simulink model "B4_quadcopter_model_discrete"  (R2021b)
settings: Solver=VariableStepAuto  StartTime=0.0  StopTime=10  FixedStep=0.002  RelTol=1e-3
values from neighbouring files (symbols this model uses):
  coef_sim_1 = tf_des_d.Denominator{1}(2)    [A11_setup_script_pprz.m]    (also in A1_setup_script.m; A6_slow_actuator.m)
  coef_sim_2 = tf_des_d.Numerator{1}(2)    [A11_setup_script_pprz.m]    (also in A1_setup_script.m; A6_slow_actuator.m)
  doublet_mag = - 0.15    (= -0.15)    [A11_setup_script_pprz.m]    (also in A1_setup_script.m)
  doublet_time = 6    [A11_setup_script_pprz.m]    (also in A1_setup_script.m)
  f_8 = 1    [A11_setup_script_pprz.m]    (also in A1_setup_script.m)
  FILT_CUTOFF = 2*pi*5    (= 31.4159265359)    [A11_setup_script_pprz.m]    (also in A1_setup_script.m)
  FILTER = 1    [A11_setup_script_pprz.m]    (also in A1_setup_script.m)
  G1 = inv(I)*G1_r    [A10_simple_plant.m]    (also in A11_setup_script_pprz.m = G1/scale; A1_setup_script.m = [G1;G1_T])
  G1_simple = inv(I)*G1_r_simple    [A1_setup_script.m]
  G2 = G2/scale    [A11_setup_script_pprz.m]    (also in A1_setup_script.m = (1/sampling_time)*inv(I)*(G2_r))
  h_plate = 0.3    [A11_setup_script_pprz.m]    (also in A1_setup_script.m = 0.16)
  I = eye(3,3)    [A10_simple_plant.m]    (also in A11_setup_script_pprz.m; A1_setup_script.m; A2_B_matrix_generation_symbolic.m = [Ixx 0 0; A3_B_matrix_generation_symbolic_cascaded.m = [Ixx 0 0)
  Iyy = 0.0008    [A11_setup_script_pprz.m]    (also in A1_setup_script.m = 0.0015)
  Izz = 0.000498    [A11_setup_script_pprz.m]    (also in A1_setup_script.m = 0.00015)
  K = 7    [A11_setup_script_pprz.m]    (also in A1_setup_script.m = 10)
  K_act = 50    [A10_simple_plant.m]    (also in A11_setup_script_pprz.m = 20; A1_setup_script.m = 20)
  K_act_outer = diag([K K K_act])    [A1_setup_script.m]
  K_d = 15    [A11_setup_script_pprz.m]    (also in A1_setup_script.m = 25)
  K_dd = K_act    (= 20)    [A11_setup_script_pprz.m]    (also in A1_setup_script.m)
  K_dyn = K    (= 10)    [A1_setup_script.m]
  K_ec = 50    [A11_setup_script_pprz.m]    (also in A1_setup_script.m = 251)
  K_ec_d = 13    [A11_setup_script_pprz.m]    (also in A1_setup_script.m = 25)
  K_ec_d_u = 1.5    [A11_setup_script_pprz.m]    (also in A1_setup_script.m = 5)
  K_ec_d_v = 1.5    [A11_setup_script_pprz.m]    (also in A1_setup_script.m = 5)
  K_ec_d_w = 1.5    [A11_setup_script_pprz.m]    (also in A1_setup_script.m = 5)
  K_ec_dd = 9    [A11_setup_script_pprz.m]    (also in A1_setup_script.m = 45)
  K_ec_i = 0    [A11_setup_script_pprz.m]    (also in A1_setup_script.m = 380)
  K_ec_u = 1.5    [A11_setup_script_pprz.m]    (also in A1_setup_script.m = 5)
  K_ec_v = 1.5    [A11_setup_script_pprz.m]    (also in A1_setup_script.m = 5)
  K_ec_w = 1.5    [A11_setup_script_pprz.m]    (also in A1_setup_script.m = 5)
  K_t = 0.0005    [A10_simple_plant.m]    (also in A11_setup_script_pprz.m = 6.557e-08; A1_setup_script.m = 6.557e-08)
  K_u = 1.0    (= 1)    [A11_setup_script_pprz.m]    (also in A1_setup_script.m = 1.5)
  K_u_d = 2.5    [A11_setup_script_pprz.m]    (also in A1_setup_script.m = 7)
  K_u_dd = K    (= 10)    [A1_setup_script.m]
  K_v = 1.0    (= 1)    [A11_setup_script_pprz.m]    (also in A1_setup_script.m = 1.5)
  K_v_d = 2.5    [A11_setup_script_pprz.m]    (also in A1_setup_script.m = 7)
  K_v_dd = K    (= 10)    [A1_setup_script.m]
  K_w = 1.0    (= 1)    [A11_setup_script_pprz.m]    (also in A1_setup_script.m = 4.5)
  K_w_d = 2.5    [A11_setup_script_pprz.m]    (also in A1_setup_script.m = 7)
  K_w_dd = K    (= 10)    [A1_setup_script.m]
  l_plate = 0.1    [A11_setup_script_pprz.m]    (also in A1_setup_script.m = 0.11)
  m = 0.4    [A10_simple_plant.m]    (also in A11_setup_script_pprz.m; A1_setup_script.m)
  NOISE = 0    [A11_setup_script_pprz.m]    (also in A1_setup_script.m)
  NOISE_ACC = 0.00005    (= 5e-05)    [A11_setup_script_pprz.m]    (also in A1_setup_script.m)
  NOISE_GYRO = 0.00005    (= 5e-05)    [A11_setup_script_pprz.m]    (also in A1_setup_script.m)
  NOISE_RPM = 200    [A11_setup_script_pprz.m]    (also in A1_setup_script.m)
  omega_act = 50    [A6_slow_actuator.m]
  omega_des = 20.00    (= 20)    [A11_setup_script_pprz.m]    (also in A1_setup_script.m; A6_slow_actuator.m = 49)
  sampling_time = 1/frequency    (= 0.002)    [A11_setup_script_pprz.m]    (also in A12_sim_multi_run.m; A1_setup_script.m; A6_slow_actuator.m)
  scale_8 = 1.6    [A11_setup_script_pprz.m]    (also in A1_setup_script.m)
  start_8 = 2    [A11_setup_script_pprz.m]    (also in A1_setup_script.m)
  start_time = 2    [A11_setup_script_pprz.m]    (also in A1_setup_script.m = 1)
  t_8 = 10    [A11_setup_script_pprz.m]    (also in A1_setup_script.m)
  w_plate = 0.3    [A11_setup_script_pprz.m]    (also in A1_setup_script.m = 0.36)
undefined symbols (not defined in the file or in its folder): DiscIntNeverNeededParam, K_ec_d_p, K_ec_d_q, K_ec_d_r, K_ec_dd_p, K_ec_dd_q, K_ec_dd_r, K_ec_i_u, K_ec_i_v, K_ec_i_w, K_ec_p, K_ec_q, K_ec_r, K_p, K_p_d, K_p_dd, K_q, K_q_d, K_q_dd, K_r, K_r_d, K_r_dd
libraries: simulink x44, cstblocks x37, dspinverses x26, dspmathops x9, dspstat3 x9, aerolibutil x9, sharedutil x3, aerolibanim x1
(part 4 of 13)

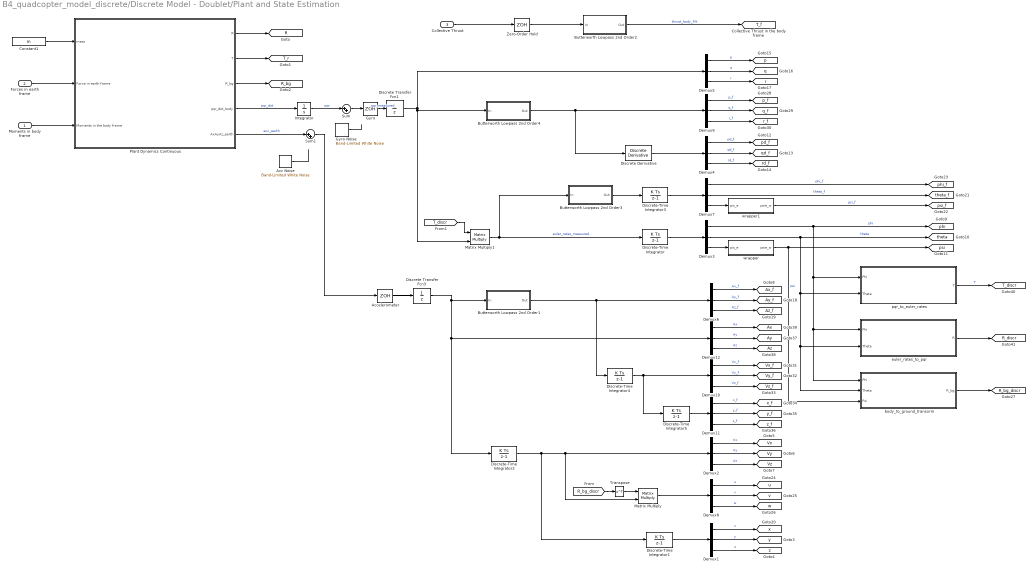
== system B4_quadcopter_model_discrete/Discrete Model - Doublet/Plant and State Estimation ==
  Moments in body frame : Inport
  Forces in earth frame : Inport  Port=2
  Collective Thrust : Inport  Port=3
  Acc Noise : simulink/Sources/Band-Limited White Noise  Cov=[NOISE_ACC]  Ts=sampling_time  seed=[23341]
  Accelerometer : ZeroOrderHold  SampleTime=sampling_time
  Butterworth Lowpass 2nd Order1 : Subsystem
  Butterworth Lowpass 2nd Order2 : Subsystem
  Butterworth Lowpass 2nd Order3 : Subsystem
  Butterworth Lowpass 2nd Order4 : Subsystem
  Constant1 : Constant  Value=m  SampleTime=sampling_time
  Demux{1..12} (12 alike) : Demux  Outputs=3
  Discrete Transfer Fcn1 : DiscreteTransferFcn  Denominator=[1 0]
  Discrete Transfer Fcn3 : DiscreteTransferFcn  Denominator=[1 0]
  Discrete Derivative : simulink/Discrete/Discrete Derivative  gainval=1.0  ICPrevScaledInput=0.0  OutMin=[]  OutMax=[]  OutDataType=fixdt(1, 16)  OutScaling=2^-10  DoSatur=off
  Discrete-Time Integrator{,1..5} (6 alike) : DiscreteIntegrator  SampleTime=sampling_time  ICPrevOutput=DiscIntNeverNeededParam  ICPrevScaledInput=DiscIntNeverNeededParam
  Gyro : ZeroOrderHold  SampleTime=sampling_time
  Gyro Noise : simulink/Sources/Band-Limited White Noise  Cov=[NOISE_GYRO]  Ts=sampling_time  seed=[23341]
  Integrator : Integrator
  Matrix Multiply : Product  Multiplication=Matrix(*)
  Matrix Multiply1 : Product  Multiplication=Matrix(*)
  Plant Dynamics Continuous : Subsystem
  Sum : Sum  Inputs=|++
  Sum1 : Sum  Inputs=|++
  Transpose : Math  Operator=transpose  SaturateOnIntegerOverflow=on
  Zero-Order Hold : ZeroOrderHold  SampleTime=sampling_time
  body_to_ground_transorm : MATLAB Function  Description=|  TreatAsAtomicUnit=on
      | This function computes the rotational matrix to pass from the body frame to the world frame. 
      | Takes as inpout the euler angles.
  euler_rates_to_pqr : MATLAB Function  TreatAsAtomicUnit=on
  pqr_to_euler_rates : MATLAB Function  TreatAsAtomicUnit=on
  wrapper : MATLAB Function  TreatAsAtomicUnit=on
  wrapper1 : MATLAB Function  TreatAsAtomicUnit=on
  tag scope: Ax=global, Ax_f=global, Ay=global, Ay_f=global, Az=global, Az_f=global, R=global, R_bg=global, R_bg_discr=global, R_discr=global, T_discr=global, T_f=global, T_r=global, Vx=global, Vx_f=global, Vy=global, Vy_f=global, Vz=global, Vz_f=global, p=global, p_f=global, pd_f=global, phi=global, phi_f=global, psi=global, psi_f=global, q=global, q_f=global, qd_f=global, r=global, r_f=global, rd_f=global, theta=global, theta_f=global, u=global, v=global, w=global, x=global, x_f=global, y=global, y_f=global, z=global, z_f=global
  wires:
  Demux3/2 -> body_to_ground_transorm/2(Theta), euler_rates_to_pqr/2(Theta), pqr_to_euler_rates/2(Theta), [theta]  "theta"
  Demux4/1 -> [pd_f]  "pd_f"
  Demux3/1 -> body_to_ground_transorm/1(Phi), euler_rates_to_pqr/1(Phi), pqr_to_euler_rates/1(Phi), [phi]  "phi"
  Demux4/2 -> [qd_f]  "qd_f"
  Demux3/3 -> wrapper/1(pis_e)
  Discrete-Time Integrator/1 -> Demux3/1
  Demux5/2 -> [q]  "q"
  Demux5/1 -> [p]  "p"
  Plant Dynamics Continuous/4(pqr_dot_body) -> Integrator/1  "pqr_dot"
  Demux5/3 -> [r]  "r"
  Integrator/1 -> Sum/1  "pqr"
  Demux4/3 -> [rd_f]  "rd_f"
  Moments in body frame/1 -> Plant Dynamics Continuous/3(Moments in the body frame)
  Constant1/1 -> Plant Dynamics Continuous/1(mass)
  Forces in earth frame/1 -> Plant Dynamics Continuous/2(Force in earth frame)
  Plant Dynamics Continuous/1(R) -> [R]
  Plant Dynamics Continuous/2(T) -> [T_r]
  Plant Dynamics Continuous/3(R_bg) -> [R_bg]
  Demux2/2 -> [Vy]  "Vy"
  Demux6/2 -> [Ay_f]  "Ay_f"
  Discrete-Time Integrator1/1 -> Demux1/1
  Demux6/1 -> [Ax_f]  "Ax_f"
  Accelerometer/1 -> Discrete Transfer Fcn3/1
  Demux2/1 -> [Vx]  "Vx"
  Demux1/2 -> [y]  "y"
  Demux1/1 -> [x]  "x"
  Demux1/3 -> [z]  "z"
  Demux6/3 -> [Az_f]  "Az_f"
  Discrete-Time Integrator2/1 -> Demux2/1, Matrix Multiply/2, Discrete-Time Integrator1/1
  Demux2/3 -> [Vz]  "Vz"
  Plant Dynamics Continuous/5(AxAyAz_earth) -> Sum1/1  "acc_earth"
  Demux7/3 -> wrapper1/1(pis_e)
  Demux7/1 -> [phi_f]  "phi_f"
  Demux7/2 -> [theta_f]  "theta_f"
  Discrete-Time Integrator3/1 -> Demux7/1
  [R_bg_discr] -> Transpose/1
  Transpose/1 -> Matrix Multiply/1
  Demux8/2 -> [v]  "v"
  Demux8/1 -> [u]  "u"
  Demux8/3 -> [w]  "w"
  Matrix Multiply/1 -> Demux8/1
  Gyro/1 -> Discrete Transfer Fcn1/1  "pqr_measured"
  Zero-Order Hold/1 -> Butterworth Lowpass 2nd Order2/1(In)
  Butterworth Lowpass 2nd Order2/1(Out) -> [T_f]  "thrust_body_filt"
  Collective Thrust/1 -> Zero-Order Hold/1
  Demux9/3 -> [r_f]  "r_f"
  Demux9/1 -> [p_f]  "p_f"
  Demux9/2 -> [q_f]  "q_f"
  Demux10/1 -> [Vx_f]  "Vx_f"
  Demux10/2 -> [Vy_f]  "Vy_f"
  Demux10/3 -> [Vz_f]  "Vz_f"
  Demux11/2 -> [y_f]  "y_f"
  Discrete-Time Integrator5/1 -> Demux11/1
  Demux11/1 -> [x_f]  "x_f"
  Demux11/3 -> [z_f]  "z_f"
  Discrete-Time Integrator4/1 -> Discrete-Time Integrator5/1, Demux10/1
  Demux12/2 -> [Ay]  "Ay"
  Demux12/1 -> [Ax]  "Ax"
  Demux12/3 -> [Az]  "Az"
  [T_discr] -> Matrix Multiply1/1
  Matrix Multiply1/1 -> Butterworth Lowpass 2nd Order3/1(In), Discrete-Time Integrator/1  "euler_rates_measured"
  Butterworth Lowpass 2nd Order3/1(Out) -> Discrete-Time Integrator3/1
  euler_rates_to_pqr/1(R) -> [R_discr]
  pqr_to_euler_rates/1(T) -> [T_discr]  "T"
  body_to_ground_transorm/1(R_bg) -> [R_bg_discr]
  Butterworth Lowpass 2nd Order1/1(Out) -> Demux6/1, Discrete-Time Integrator4/1
  wrapper/1(psie_w) -> body_to_ground_transorm/3(Psi), [psi]  "psi"
  wrapper1/1(psie_w) -> [psi_f]  "psi_f"
  Sum/1 -> Gyro/1
  Gyro Noise/1 -> ?
  Acc Noise/1 -> ?
  Sum1/1 -> Accelerometer/1
  Discrete Transfer Fcn1/1 -> Demux5/1, Butterworth Lowpass 2nd Order4/1(In), Matrix Multiply1/2
  Discrete Derivative/1 -> Demux4/1
  Discrete Transfer Fcn3/1 -> Discrete-Time Integrator2/1, Demux12/1, Butterworth Lowpass 2nd Order1/1(In)
  Butterworth Lowpass 2nd Order4/1(Out) -> Demux9/1, Discrete Derivative/1

== system B4_quadcopter_model_discrete/Discrete Model - Inner Loop Only/Continuous Actuator Dynamics ==
  Motor_1_omega_input : Inport
  Motor_2_omega_input : Inport  Port=2
  Motor_3_omega_input : Inport  Port=3
  Motor_4_omega_input : Inport  Port=4
  Butterworth Lowpass 2nd Order1 : Subsystem
  Demux : Demux
  Discrete Transfer Fcn{1..4} (4 alike) : DiscreteTransferFcn  Numerator=[coef_sim_2]  Denominator=[1 coef_sim_1]  SampleTime=sampling_time
  Mux : Mux
  RPM Noise : simulink/Sources/Band-Limited White Noise  Cov=[NOISE_RPM]  Ts=sampling_time  seed=[23341]
  Saturation{,1..3} (4 alike) : Saturate  UpperLimit=12000  LowerLimit=0
  Sum : Sum  Inputs=|++
  Transfer Fcn{,1..3} (4 alike) : TransferFcn  Numerator=[omega_des]  Denominator=[1 omega_des]
  omega_1 : Outport
  omega_2 : Outport  Port=2
  omega_3 : Outport  Port=3
  omega_4 : Outport  Port=4
  tag scope: omega_1_f=global, omega_2_f=global, omega_3_f=global, omega_4_f=global
  wires:
  Transfer Fcn3/1 -> omega_4/1  "omega_4"
  Motor_4_omega_input/1 -> Saturation3/1  "omega_4_in"
  Saturation/1 -> Discrete Transfer Fcn2/1, Transfer Fcn/1
  Motor_3_omega_input/1 -> Saturation2/1  "omega_3_in"
  Transfer Fcn1/1 -> omega_2/1  "omega_2"
  Saturation1/1 -> Transfer Fcn1/1, Discrete Transfer Fcn1/1
  Saturation3/1 -> Transfer Fcn3/1, Discrete Transfer Fcn4/1
  Discrete Transfer Fcn2/1 -> Mux/1
  Saturation2/1 -> Transfer Fcn2/1, Discrete Transfer Fcn3/1
  Motor_2_omega_input/1 -> Saturation1/1  "omega_2_in"
  Demux/2 -> [omega_2_f]  "omega_2_est"
  Motor_1_omega_input/1 -> Saturation/1  "omega_1_in"
  Transfer Fcn/1 -> omega_1/1  "omega_1"
  Demux/4 -> [omega_4_f]  "omega_4_est"
  Discrete Transfer Fcn4/1 -> Mux/4
  Discrete Transfer Fcn1/1 -> Mux/2
  Discrete Transfer Fcn3/1 -> Mux/3
  Transfer Fcn2/1 -> omega_3/1  "omega_3"
  Demux/1 -> [omega_1_f]  "omega_1_est"
  Demux/3 -> [omega_3_f]  "omega_3_est"
  Mux/1 -> Sum/1
  Butterworth Lowpass 2nd Order1/1(Out) -> Demux/1
  RPM Noise/1 -> ?
  Sum/1 -> Butterworth Lowpass 2nd Order1/1(In)

== system B4_quadcopter_model_discrete/Discrete Model - Inner Loop Only/Discrete INDI Controller Cascaded ==
  note: Inner Loop
  Constant : Constant  Value=0
  Constant2 : Constant  Value=G1  SampleTime=sampling_time
  Constant3 : Constant  Value=G2  SampleTime=sampling_time
  Constant9 : Constant  Value=G2  SampleTime=sampling_time
  Demux : Demux
  Demux1 : Demux  Outputs=3
  Discrete Transfer Fcn : DiscreteTransferFcn  Denominator=[1 0]
  Display : Display
  Doublet Block : Subsystem
  ERROR CONTROLLER ATTITUDE : Subsystem
  G1+G2 : MATLAB Function  TreatAsAtomicUnit=on
  G2_comp : MATLAB Function  TreatAsAtomicUnit=on
  INTERNAL REFERENCE MODEL ATTITUDE : Subsystem
  Matrix Multiply : Product  Multiplication=Matrix(*)
  Pseudoinverse2 : dspinverses/Pseudoinverse  wanterr=off  SimulateUsing=Interpreted execution
      settings: SourceProductBaseCode=DS
  Saturation4 : Saturate  UpperLimit=12000  LowerLimit=10
  Scope1 : Scope
  Sum{,4..5,8,11,13} (6 alike) : Sum  Inputs=|++
  Sum1 : Sum  Inputs=|+-
  Sum2 : Sum  Inputs=|+-
  Sum3 : Sum  Inputs=|+-
  Vector Concatenate : Concatenate  NumInputs=3
  Vector Concatenate1 : Concatenate  NumInputs=4
  Vector Concatenate2 : Concatenate  NumInputs=3
  Motor_1_omega_input : Outport
  Motor_2_omega_input : Outport  Port=2
  Motor_3_omega_input : Outport  Port=3
  Motor_4_omega_input : Outport  Port=4
  wires:
  Sum13/1 -> Sum3/1  "rd_des"
  Sum4/1 -> Sum1/1  "pd_des"
  Sum2/1 -> Vector Concatenate/2
  ERROR CONTROLLER ATTITUDE/1(pd_ec) -> Sum4/2  "pd_ec"
  Sum3/1 -> Vector Concatenate/3
  ERROR CONTROLLER ATTITUDE/3(rd_ec) -> Sum13/2  "rd_ec"
  INTERNAL REFERENCE MODEL ATTITUDE/5(q_ref) -> ERROR CONTROLLER ATTITUDE/2(q_ref)  "q_ref"
  Vector Concatenate/1 -> [dv_inner], Scope1/1
  [pd_f] -> Sum1/2
  INTERNAL REFERENCE MODEL ATTITUDE/3(rd_ref) -> Sum13/1  "rd_ref"
  INTERNAL REFERENCE MODEL ATTITUDE/9(psi_ref) -> ERROR CONTROLLER ATTITUDE/6(psi_ref)  "psi_ref"
  INTERNAL REFERENCE MODEL ATTITUDE/4(p_ref) -> ERROR CONTROLLER ATTITUDE/1(p_ref)  "p_ref"
  INTERNAL REFERENCE MODEL ATTITUDE/6(r_ref) -> ERROR CONTROLLER ATTITUDE/3(r_ref)  "r_ref"
  INTERNAL REFERENCE MODEL ATTITUDE/8(theta_ref) -> ERROR CONTROLLER ATTITUDE/5(theta_ref)  "theta_ref"
  INTERNAL REFERENCE MODEL ATTITUDE/7(phi_ref) -> ERROR CONTROLLER ATTITUDE/4(phi_ref)  "phi_ref"
  ERROR CONTROLLER ATTITUDE/2(qd_ec) -> Sum11/2  "qd_ec"
  INTERNAL REFERENCE MODEL ATTITUDE/1(pd_ref) -> Sum4/1  "pd_ref"
  Sum1/1 -> Vector Concatenate/1
  Sum11/1 -> Sum2/1  "qd_des"
  [qd_f] -> Sum2/2
  INTERNAL REFERENCE MODEL ATTITUDE/2(qd_ref) -> Sum11/1  "qd_ref"
  [rd_f] -> Sum3/2
  Saturation4/1 -> Discrete Transfer Fcn/1
  Demux/4 -> Motor_4_omega_input/1
  Pseudoinverse2/1 -> Matrix Multiply/1
  Vector Concatenate2/1 -> Matrix Multiply/2
  Constant9/1 -> G2_comp/1(G2)
  Sum/1 -> Vector Concatenate2/3
  Demux1/3 -> Sum/1
  Demux1/2 -> Vector Concatenate2/2
  Constant2/1 -> G1+G2/1(G1)
  Discrete Transfer Fcn/1 -> G2_comp/2(domega)
  Constant3/1 -> G1+G2/2(G2)
  Demux/3 -> Motor_3_omega_input/1
  [omega_1_f] -> Vector Concatenate1/1
  Vector Concatenate1/1 -> Sum8/2  "u"
  G2_comp/1(G2_comp) -> Sum/2  "G2_comp"
  Demux1/1 -> Vector Concatenate2/1
  Matrix Multiply/1 -> Saturation4/1, Sum8/1  "du"
  Demux/1 -> Motor_1_omega_input/1
  [omega_3_f] -> Vector Concatenate1/3
  Sum8/1 -> Demux/1  "u_cmd"
  Demux/2 -> Motor_2_omega_input/1
  [omega_2_f] -> Vector Concatenate1/2
  G1+G2/1(B_inner) -> Pseudoinverse2/1, Display/1  "B_inner"
  [dv_inner] -> Demux1/1  "dv_inner"
  [omega_4_f] -> Vector Concatenate1/4
  Constant/1 -> INTERNAL REFERENCE MODEL ATTITUDE/1(phi_cmd), Sum5/1  "phi_cmd"
  Sum5/1 -> INTERNAL REFERENCE MODEL ATTITUDE/2(theta_cmd)  "theta_cmd"
  Doublet Block/1(Out1) -> Sum5/2

== system B4_quadcopter_model_discrete/Discrete Model - Inner Loop Only/Discrete INDI Controller Cascaded w// Actuator Compensation ==
  Constant : Constant  Value=0
  Constant2 : Constant  Value=G1_simple  SampleTime=sampling_time
  Constant6 : Constant  Value=K_act  SampleTime=sampling_time
  Demux : Demux
  Display : Display
  Doublet Block : Subsystem
  ERROR CONTROLLER ATTITUDE : Subsystem
  G1+G2 : MATLAB Function  TreatAsAtomicUnit=on
  INTERNAL REFERENCE MODEL ATTITUDE : Subsystem
  Matrix Multiply : Product  Multiplication=Matrix(*)
  Pseudoinverse2 : dspinverses/Pseudoinverse  wanterr=off  SimulateUsing=Interpreted execution
      settings: SourceProductBaseCode=DS
  Sum{1,4,8,11,13} (5 alike) : Sum  Inputs=|++
  Vector Concatenate : Concatenate  NumInputs=3
  Vector Concatenate1 : Concatenate  NumInputs=4
  Motor_1_omega_input : Outport
  Motor_2_omega_input : Outport  Port=2
  Motor_3_omega_input : Outport  Port=3
  Motor_4_omega_input : Outport  Port=4
  wires:
  G1+G2/1(B_inner) -> Pseudoinverse2/1, Display/1  "B_inner"
  Vector Concatenate1/1 -> Sum8/2  "u"
  Vector Concatenate/1 -> [dv_inner]
  Matrix Multiply/1 -> Sum8/1  "du"
  Demux/1 -> Motor_1_omega_input/1
  [omega_4_f] -> Vector Concatenate1/4
  [omega_2_f] -> Vector Concatenate1/2
  Demux/3 -> Motor_3_omega_input/1
  Sum8/1 -> Demux/1  "u_cmd"
  Pseudoinverse2/1 -> Matrix Multiply/1
  [omega_1_f] -> Vector Concatenate1/1
  Demux/2 -> Motor_2_omega_input/1
  Demux/4 -> Motor_4_omega_input/1
  [omega_3_f] -> Vector Concatenate1/3
  INTERNAL REFERENCE MODEL ATTITUDE/4(pd_ref) -> ERROR CONTROLLER ATTITUDE/1(pd_ref)
  INTERNAL REFERENCE MODEL ATTITUDE/7(p_ref) -> ERROR CONTROLLER ATTITUDE/4(p_ref)
  ERROR CONTROLLER ATTITUDE/3(rdd_ec) -> Sum13/2  "rdd_ec"
  ERROR CONTROLLER ATTITUDE/2(qdd_ec) -> Sum11/2  "qdd_ec"
  INTERNAL REFERENCE MODEL ATTITUDE/5(qd_ref) -> ERROR CONTROLLER ATTITUDE/2(qd_ref)
  INTERNAL REFERENCE MODEL ATTITUDE/11(theta_ref) -> ERROR CONTROLLER ATTITUDE/8(theta_ref)
  INTERNAL REFERENCE MODEL ATTITUDE/1(pdd_ref) -> Sum4/1
  INTERNAL REFERENCE MODEL ATTITUDE/3(rdd_ref) -> Sum13/1
  INTERNAL REFERENCE MODEL ATTITUDE/8(q_ref) -> ERROR CONTROLLER ATTITUDE/5(q_ref)
  ERROR CONTROLLER ATTITUDE/1(pdd_ec) -> Sum4/2  "pdd_ec"
  INTERNAL REFERENCE MODEL ATTITUDE/6(rd_ref) -> ERROR CONTROLLER ATTITUDE/3(rd_ref)
  INTERNAL REFERENCE MODEL ATTITUDE/10(phi_ref) -> ERROR CONTROLLER ATTITUDE/7(phi_ref)
  INTERNAL REFERENCE MODEL ATTITUDE/12(psi_ref) -> ERROR CONTROLLER ATTITUDE/9(psi_ref)
  INTERNAL REFERENCE MODEL ATTITUDE/9(r_ref) -> ERROR CONTROLLER ATTITUDE/6(r_ref)
  Sum13/1 -> Vector Concatenate/3  "rdd_des"
  Sum4/1 -> Vector Concatenate/1  "pdd_des"
  Sum11/1 -> Vector Concatenate/2  "qdd_des"
  Constant6/1 -> G1+G2/2(K_act)
  Constant2/1 -> G1+G2/1(G1_simple)
  [dv_inner] -> Matrix Multiply/2  "dv_inner"
  INTERNAL REFERENCE MODEL ATTITUDE/2(qdd_ref) -> Sum11/1
  Constant/1 -> INTERNAL REFERENCE MODEL ATTITUDE/3(psi_cmd), INTERNAL REFERENCE MODEL ATTITUDE/1(phi_cmd), Sum1/1  "phi_cmd"
  Sum1/1 -> INTERNAL REFERENCE MODEL ATTITUDE/2(theta_cmd)  "theta_cmd"
  Doublet Block/1(Out1) -> Sum1/2

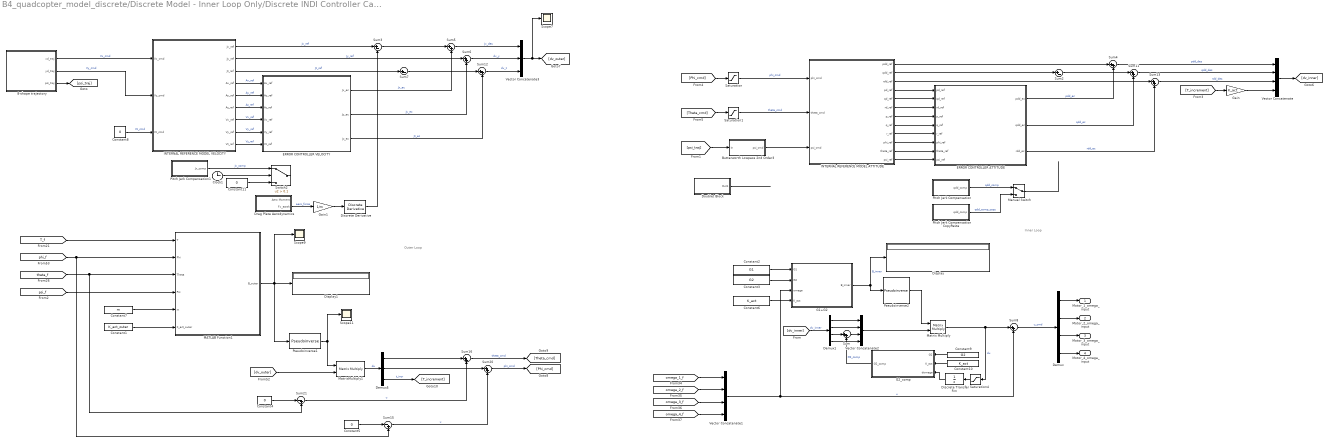
== system B4_quadcopter_model_discrete/Discrete Model - Inner Loop Only/Discrete INDI Controller Cascaded w// Actuator Compensation Double ==
  note: Outer Loop
  note: Inner Loop
  8-shape trajectory : Subsystem
  Butterworth Lowpass 2nd Order3 : Subsystem
  Clock1 : Clock
      settings: Decimation=100
  Constant1 : Constant  Value=K_act_outer  SampleTime=sampling_time
  Constant10 : Constant  Value=K_act  SampleTime=sampling_time
  Constant11 : Constant  Value=0
  Constant2 : Constant  Value=G1  SampleTime=sampling_time
  Constant3 : Constant  Value=G2  SampleTime=sampling_time
  Constant4 : Constant  Value=0
  Constant5 : Constant  Value=0
  Constant6 : Constant  Value=K_act  SampleTime=sampling_time
  Constant7 : Constant  Value=m  SampleTime=sampling_time
  Constant8 : Constant  Value=0  SampleTime=sampling_time
  Constant9 : Constant  Value=G2  SampleTime=sampling_time
  Demux : Demux
  Demux1 : Demux
  Demux5 : Demux  Outputs=3
  Discrete Transfer Fcn : DiscreteTransferFcn  Denominator=[1 0]
  Discrete Derivative : simulink/Discrete/Discrete Derivative  gainval=1.0  ICPrevScaledInput=0.0  OutMin=[]  OutMax=[]  OutDataType=fixdt(1, 16)  OutScaling=2^-10  DoSatur=off
  Display : Display
  Display1 : Display
  Doublet Block : Subsystem
  Drag Plate Aerodynamics : Subsystem
  ERROR CONTROLLER ATTITUDE : Subsystem
  ERROR CONTROLLER VELOCITY : Subsystem
  G1+G2 : MATLAB Function  TreatAsAtomicUnit=on
  G2_comp : MATLAB Function  TreatAsAtomicUnit=on
  Gain : Gain  Gain=K_act
  Gain1 : Gain  Gain=1/m
  INTERNAL REFERENCE MODEL ATTITUDE : Subsystem
  INTERNAL REFERENCE MODEL VELOCITY : Subsystem
  MATLAB Function1 : MATLAB Function  TreatAsAtomicUnit=on
  Manual Switch : ManualSwitch
  Matrix Multiply : Product  Multiplication=Matrix(*)
  MatrixMultiply1 : Product  Multiplication=Matrix(*)
  Pitch Jerk Compensation : Subsystem
  Pitch Jerk Compensation CopyPaste : Subsystem
  Pitch Jerk Compensation1 : Subsystem
  Pseudoinverse1 : dspinverses/Pseudoinverse  wanterr=off  SimulateUsing=Interpreted execution
      settings: SourceProductBaseCode=DS
  Pseudoinverse2 : dspinverses/Pseudoinverse  wanterr=off  SimulateUsing=Interpreted execution
      settings: SourceProductBaseCode=DS
  Saturation : Saturate
  Saturation1 : Saturate
  Saturation4 : Saturate  UpperLimit=12000  LowerLimit=10
  Scope11 : Scope
  Scope7 : Scope
  Scope9 : Scope
  Sum{,4..6,8,11..13,16,20} (10 alike) : Sum  Inputs=|++
  Sum15 : Sum  Inputs=|-+
  Sum2 : Sum  Inputs=|+-
  Sum21 : Sum  Inputs=|-+
  Sum3 : Sum  Inputs=|+-
  Sum7 : Sum  Inputs=|+-
  Switch2 : Switch  Criteria=u2 > Threshold  Threshold=0.1
  Vector Concatenate : Concatenate  NumInputs=4
  Vector Concatenate1 : Concatenate  NumInputs=4
  Vector Concatenate2 : Concatenate  NumInputs=4
  Vector Concatenate3 : Concatenate  NumInputs=3
  Motor_1_omega_input : Outport
  Motor_2_omega_input : Outport  Port=2
  Motor_3_omega_input : Outport  Port=3
  Motor_4_omega_input : Outport  Port=4
  wires:
  Constant4/1 -> Sum21/1
  Sum16/1 -> [Theta_cmd]  "theta_cmd"
  Sum12/1 -> Vector Concatenate3/3  "dv_z"
  INTERNAL REFERENCE MODEL VELOCITY/2(Jy_ref) -> Sum6/1  "Jy_ref"
  Sum21/1 -> Sum16/2  "u"
  ERROR CONTROLLER VELOCITY/2(Jy_ec) -> Sum6/2  "Jy_ec"
  8-shape trajectory/1(xd_traj) -> INTERNAL REFERENCE MODEL VELOCITY/1(Vx_cmd)  "Vx_cmd"
  Sum6/1 -> Vector Concatenate3/2  "dv_y"
  ERROR CONTROLLER VELOCITY/1(Jx_ec) -> Sum5/2  "Jx_ec"
  Sum5/1 -> Vector Concatenate3/1  "Jx_des"
  ERROR CONTROLLER VELOCITY/3(Jz_ec) -> Sum12/2  "Jz_ec"
  Constant8/1 -> INTERNAL REFERENCE MODEL VELOCITY/3(Vz_cmd)  "Vz_cmd"
  Pseudoinverse1/1 -> Scope11/1, MatrixMultiply1/1
  Sum15/1 -> Sum20/2  "u"
  Vector Concatenate3/1 -> Scope7/1, [dv_outer]
  INTERNAL REFERENCE MODEL VELOCITY/1(Jx_ref) -> Sum3/1  "Jx_ref"
  INTERNAL REFERENCE MODEL VELOCITY/3(Jz_ref) -> Sum7/1  "Jz_ref"
  Sum20/1 -> [Phi_cmd]  "phi_cmd"
  [T_f] -> MATLAB Function1/1(T)
  Constant7/1 -> MATLAB Function1/5(m)
  Constant5/1 -> Sum15/1
  [dv_outer] -> MatrixMultiply1/2
  Demux5/1 -> Sum16/1
  MATLAB Function1/1(B_outer) -> Pseudoinverse1/1, Display1/1, Scope9/1
  Demux5/3 -> [T_increment]  "t_incr"
  MatrixMultiply1/1 -> Demux5/1  "du"
  Demux5/2 -> Sum20/1
  8-shape trajectory/2(yd_traj) -> INTERNAL REFERENCE MODEL VELOCITY/2(Vy_cmd)  "Vy_cmd"
  [theta_f] -> Sum21/2, MATLAB Function1/3(Theta)
  [phi_f] -> Sum15/2, MATLAB Function1/2(Phi)
  8-shape trajectory/3(psi_traj) -> [psi_traj]
  INTERNAL REFERENCE MODEL VELOCITY/4(Ax_ref) -> ERROR CONTROLLER VELOCITY/1(Ax_ref)  "Ax_ref"
  INTERNAL REFERENCE MODEL VELOCITY/5(Ay_ref) -> ERROR CONTROLLER VELOCITY/2(Ay_ref)  "Ay_ref"
  INTERNAL REFERENCE MODEL VELOCITY/6(Az_ref) -> ERROR CONTROLLER VELOCITY/3(Az_ref)  "Az_ref"
  INTERNAL REFERENCE MODEL VELOCITY/7(Vx_ref) -> ERROR CONTROLLER VELOCITY/4(Vx_ref)  "Vx_ref"
  INTERNAL REFERENCE MODEL VELOCITY/8(Vy_ref) -> ERROR CONTROLLER VELOCITY/5(Vy_ref)  "Vy_ref"
  INTERNAL REFERENCE MODEL VELOCITY/9(Vz_ref) -> ERROR CONTROLLER VELOCITY/6(Vz_ref)  "Vz_ref"
  Sum3/1 -> Sum5/1
  Sum7/1 -> Sum12/1
  Constant1/1 -> MATLAB Function1/6(K_act_outer)
  [psi_f] -> MATLAB Function1/4(Psi)
  INTERNAL REFERENCE MODEL ATTITUDE/12(psi_ref) -> ERROR CONTROLLER ATTITUDE/9(psi_ref)
  Demux1/1 -> Vector Concatenate2/1
  ERROR CONTROLLER ATTITUDE/2(qdd_ec) -> Sum11/2  "qdd_ec"
  Sum4/1 -> Vector Concatenate/1  "pdd_des"
  [dv_inner] -> Demux1/1  "dv_inner"
  Demux1/4 -> Vector Concatenate2/4
  INTERNAL REFERENCE MODEL ATTITUDE/3(rdd_ref) -> Sum13/1
  Sum2/1 -> Sum11/1
  INTERNAL REFERENCE MODEL ATTITUDE/9(r_ref) -> ERROR CONTROLLER ATTITUDE/6(r_ref)
  [omega_2_f] -> Vector Concatenate1/2
  Sum11/1 -> Vector Concatenate/2  "qdd_des"
  INTERNAL REFERENCE MODEL ATTITUDE/10(phi_ref) -> ERROR CONTROLLER ATTITUDE/7(phi_ref)
  Demux1/2 -> Vector Concatenate2/2
  G2_comp/1(G2_comp) -> Sum/2  "G2_comp"
  Saturation1/1 -> INTERNAL REFERENCE MODEL ATTITUDE/2(theta_cmd)  "theta_cmd"
  [Theta_cmd] -> Saturation1/1
  Demux/3 -> Motor_3_omega_input/1
  INTERNAL REFERENCE MODEL ATTITUDE/4(pd_ref) -> ERROR CONTROLLER ATTITUDE/1(pd_ref)
  Saturation/1 -> INTERNAL REFERENCE MODEL ATTITUDE/1(phi_cmd)  "phi_cmd"
  Doublet Block/1(Out1) -> ?
  INTERNAL REFERENCE MODEL ATTITUDE/7(p_ref) -> ERROR CONTROLLER ATTITUDE/4(p_ref)
  Sum/1 -> Vector Concatenate2/3
  Demux1/3 -> Sum/1
  [omega_1_f] -> Vector Concatenate1/1
  INTERNAL REFERENCE MODEL ATTITUDE/2(qdd_ref) -> Sum2/1
  INTERNAL REFERENCE MODEL ATTITUDE/11(theta_ref) -> ERROR CONTROLLER ATTITUDE/8(theta_ref)
  Constant3/1 -> G1+G2/2(G2)
  Vector Concatenate1/1 -> G1+G2/3(omega), Sum8/2  "u"
  Saturation4/1 -> Discrete Transfer Fcn/1
  Pseudoinverse2/1 -> Matrix Multiply/1
  Demux/4 -> Motor_4_omega_input/1
  Butterworth Lowpass 2nd Order3/1(psi_cmd) -> INTERNAL REFERENCE MODEL ATTITUDE/3(psi_cmd)
  Sum13/1 -> Vector Concatenate/3  "rdd_des"
  Vector Concatenate2/1 -> Matrix Multiply/2
  ERROR CONTROLLER ATTITUDE/3(rdd_ec) -> Sum13/2  "rdd_ec"
  Constant10/1 -> G2_comp/2(K_act)
  [omega_4_f] -> Vector Concatenate1/4
  ERROR CONTROLLER ATTITUDE/1(pdd_ec) -> Sum4/2  "pdd_ec"
  Discrete Transfer Fcn/1 -> G2_comp/3(domega)
  INTERNAL REFERENCE MODEL ATTITUDE/8(q_ref) -> ERROR CONTROLLER ATTITUDE/5(q_ref)
  Pitch Jerk Compensation CopyPaste/1(qdd_comp) -> Manual Switch/2  "qdd_comp_copy"
  Demux/2 -> Motor_2_omega_input/1
  Constant2/1 -> G1+G2/1(G1)
  Constant9/1 -> G2_comp/1(G2)
  INTERNAL REFERENCE MODEL ATTITUDE/1(pdd_ref) -> Sum4/1
  G1+G2/1(B_inner) -> Pseudoinverse2/1, Display/1  "B_inner"
  [T_increment] -> Gain/1
  Demux/1 -> Motor_1_omega_input/1
  [psi_traj] -> Butterworth Lowpass 2nd Order3/1(In)
  Constant6/1 -> G1+G2/4(K_act)
  INTERNAL REFERENCE MODEL ATTITUDE/6(rd_ref) -> ERROR CONTROLLER ATTITUDE/3(rd_ref)
  Manual Switch/1 -> ?
  Vector Concatenate/1 -> [dv_inner]
  Sum8/1 -> Demux/1  "u_cmd"
  [omega_3_f] -> Vector Concatenate1/3
  INTERNAL REFERENCE MODEL ATTITUDE/5(qd_ref) -> ERROR CONTROLLER ATTITUDE/2(qd_ref)
  Gain/1 -> Vector Concatenate/4
  [Phi_cmd] -> Saturation/1
  Matrix Multiply/1 -> Saturation4/1, Sum8/1  "du"
  Pitch Jerk Compensation/1(qdd_comp) -> Manual Switch/1  "qdd_comp"
  Constant11/1 -> Switch2/3
  Pitch Jerk Compensation1/1(Jx_comp) -> Switch2/1  "Jx_comp"
  Clock1/1 -> Switch2/2
  Drag Plate Aerodynamics/2(Fx_earth) -> Gain1/1  "aero_force"
  Gain1/1 -> Discrete Derivative/1
  Discrete Derivative/1 -> Sum3/2

== system B4_quadcopter_model_discrete/Discrete Model - Inner Loop Only/Force and Moment Calculation ==
  omega_1 : Inport
  omega_2 : Inport  Port=2
  omega_3 : Inport  Port=3
  omega_4 : Inport  Port=4
  Constant2 : Constant  Value=G1_simple  SampleTime=sampling_time
  Constant5 : Constant  Value=I  SampleTime=sampling_time
  Moments due to thrust : MATLAB Function  TreatAsAtomicUnit=on
  Mux : Mux
  Moments in body frame : Outport
  wires:
  Constant2/1 -> Moments due to thrust/2(G1_simple)
  omega_4/1 -> Mux/4
  omega_3/1 -> Mux/3
  omega_2/1 -> Mux/2
  omega_1/1 -> Mux/1
  Mux/1 -> Moments due to thrust/1(omega)
  Moments due to thrust/1(M_t) -> Moments in body frame/1  "total_moment"
  Constant5/1 -> Moments due to thrust/3(I)

== system B4_quadcopter_model_discrete/Discrete Model - Inner Loop Only/Plant and State Estimation ==
  Moments in body frame : Inport
  Butterworth Lowpass 2nd Order3 : Subsystem
  Butterworth Lowpass 2nd Order4 : Subsystem
  Butterworth Lowpass 2nd Order5 : Subsystem
  Demux{3..5,7,9} (5 alike) : Demux  Outputs=3
  Discrete Derivative : simulink/Discrete/Discrete Derivative  gainval=1.0  ICPrevScaledInput=0.0  OutMin=[]  OutMax=[]  OutDataType=fixdt(1, 16)  OutScaling=2^-10  DoSatur=off
  Discrete-Time Integrator : DiscreteIntegrator  SampleTime=sampling_time  ICPrevOutput=DiscIntNeverNeededParam  ICPrevScaledInput=DiscIntNeverNeededParam
  Discrete-Time Integrator3 : DiscreteIntegrator  SampleTime=sampling_time  ICPrevOutput=DiscIntNeverNeededParam  ICPrevScaledInput=DiscIntNeverNeededParam
  Gyro : ZeroOrderHold  SampleTime=sampling_time
  Gyro Noise : simulink/Sources/Band-Limited White Noise  Cov=[NOISE_GYRO]  Ts=sampling_time  seed=[23341]
  Integrator : Integrator
  Plant Dynamics Continuous : Subsystem
  Sum : Sum  Inputs=|++
  wrapper : MATLAB Function  TreatAsAtomicUnit=on
  wrapper1 : MATLAB Function  TreatAsAtomicUnit=on
  tag scope: p=global, p_f=global, pd_f=global, phi=global, phi_f=global, psi=global, psi_f=global, q=global, q_f=global, qd_f=global, r=global, r_f=global, rd_f=global, theta=global, theta_f=global
  wires:
  Demux3/2 -> [theta]  "theta"
  Demux4/1 -> [pd_f]  "pd_f"
  Demux3/1 -> [phi]  "phi"
  Demux4/2 -> [qd_f]  "qd_f"
  Demux3/3 -> wrapper/1(pis_e)
  Discrete-Time Integrator/1 -> Demux3/1
  Demux5/2 -> [q]  "q"
  Demux5/1 -> [p]  "p"
  Plant Dynamics Continuous/1(pqr_dot_body) -> Integrator/1  "pqr_dot"
  Demux5/3 -> [r]  "r"
  Integrator/1 -> Sum/1  "pqr"
  Discrete Derivative/1 -> Butterworth Lowpass 2nd Order4/1(In)
  Demux4/3 -> [rd_f]  "rd_f"
  Moments in body frame/1 -> Plant Dynamics Continuous/1(Moments in the body frame)
  Demux7/3 -> wrapper1/1(pis_e)
  Demux7/1 -> [phi_f]  "phi_f"
  Demux7/2 -> [theta_f]  "theta_f"
  Discrete-Time Integrator3/1 -> Demux7/1
  Gyro/1 -> Discrete Derivative/1, Butterworth Lowpass 2nd Order5/1(In), Butterworth Lowpass 2nd Order3/1(In), Discrete-Time Integrator/1, Demux5/1  "pqr_measured"
  Demux9/3 -> [r_f]  "r_f"
  Demux9/1 -> [p_f]  "p_f"
  Demux9/2 -> [q_f]  "q_f"
  Butterworth Lowpass 2nd Order3/1(Out) -> Discrete-Time Integrator3/1
  wrapper/1(psie_w) -> [psi]  "psi"
  wrapper1/1(psie_w) -> [psi_f]  "psi_f"
  Sum/1 -> Gyro/1
  Gyro Noise/1 -> ?
  Butterworth Lowpass 2nd Order5/1(Out) -> Demux9/1
  Butterworth Lowpass 2nd Order4/1(Out) -> Demux4/1

== system B4_quadcopter_model_discrete/Discrete Model - Oversimplified/Butterworth Lowpass 2nd Order1 ==
  In : Inport
  Constant : Constant  Value=FILTER  SampleTime=sampling_time
  Merge : Merge
  Switch Case : SwitchCase
  Switch Case Action Subsystem : Subsystem  TreatAsAtomicUnit=on
  Switch Case Action Subsystem1 : Subsystem  TreatAsAtomicUnit=on
  Out : Outport
  wires:
  Merge/1 -> Out/1
  Switch Case Action Subsystem/1(Out1) -> Merge/1
  Constant/1 -> Switch Case/1
  Switch Case Action Subsystem1/1(Out1) -> Merge/2
  Switch Case/2 -> Switch Case Action Subsystem1/Action
  In/1 -> Switch Case Action Subsystem/1(In1), Switch Case Action Subsystem1/1(In1)
  Switch Case/1 -> Switch Case Action Subsystem/Action

== system B4_quadcopter_model_discrete/Discrete Model - Oversimplified/Butterworth Lowpass 2nd Order4 ==
  In : Inport
  Constant : Constant  Value=FILTER  SampleTime=sampling_time
  Merge : Merge
  Switch Case : SwitchCase
  Switch Case Action Subsystem : Subsystem  TreatAsAtomicUnit=on
  Switch Case Action Subsystem1 : Subsystem  TreatAsAtomicUnit=on
  Out : Outport
  wires:
  Merge/1 -> Out/1
  Switch Case Action Subsystem/1(Out1) -> Merge/1
  Constant/1 -> Switch Case/1
  Switch Case Action Subsystem1/1(Out1) -> Merge/2
  Switch Case/2 -> Switch Case Action Subsystem1/Action
  In/1 -> Switch Case Action Subsystem/1(In1), Switch Case Action Subsystem1/1(In1)
  Switch Case/1 -> Switch Case Action Subsystem/Action

== system B4_quadcopter_model_discrete/Discrete Model - Oversimplified/Doublet Block ==
  Scope : Scope
  Step : Step  Time=start_time  After=doublet_mag  SampleTime=sampling_time
  Step1 : Step  Time=start_time + doublet_time/2  After=-doublet_mag  SampleTime=sampling_time
  Step2 : Step  Time=start_time + doublet_time  After=0  SampleTime=sampling_time
  Sum : Sum  Inputs=|++
  Sum1 : Sum  Inputs=|++
  Out1 : Outport
  wires:
  Step1/1 -> Sum/2
  Sum/1 -> Sum1/1
  Sum1/1 -> Out1/1, Scope/1
  Step2/1 -> Sum1/2
  Step/1 -> Sum/1

== system B4_quadcopter_model_discrete/Discrete Model - Oversimplified/Doublet Block1 ==
  Scope : Scope
  Step : Step  Time=start_time  After=doublet_mag  SampleTime=sampling_time
  Step1 : Step  Time=start_time + doublet_time/2  After=-doublet_mag  SampleTime=sampling_time
  Step2 : Step  Time=start_time + doublet_time  After=0  SampleTime=sampling_time
  Sum : Sum  Inputs=|++
  Sum1 : Sum  Inputs=|++
  Out1 : Outport
  wires:
  Step1/1 -> Sum/2
  Sum/1 -> Sum1/1
  Sum1/1 -> Out1/1, Scope/1
  Step2/1 -> Sum1/2
  Step/1 -> Sum/1

== system B4_quadcopter_model_discrete/Discrete Model - Oversimplified/ERROR CONTROLLER ATTITUDE ==
  pd_ref : Inport
  qd_ref : Inport  Port=2
  rd_ref : Inport  Port=3
  p_ref : Inport  Port=4
  q_ref : Inport  Port=5
  r_ref : Inport  Port=6
  phi_ref : Inport  Port=7
  theta_ref : Inport  Port=8
  psi_ref : Inport  Port=9
  Add : Sum  Inputs=+++
  Add1 : Sum  Inputs=+++
  Add2 : Sum  Inputs=+++
  Gain : Gain  Gain=K_ec_dd_p + K_act
  Gain1 : Gain  Gain=K_ec_d_p *(1 + K_act)
  Gain2 : Gain  Gain=K_ec_p *(1 + K_act)
  Gain3 : Gain  Gain=K_ec_dd_q + K_act
  Gain4 : Gain  Gain=K_ec_d_q *(1 + K_act)
  Gain5 : Gain  Gain=K_ec_q *(1 + K_act)
  Gain6 : Gain  Gain=K_ec_dd_r + K_act
  Gain7 : Gain  Gain=K_ec_d_r *(1 + K_act)
  Gain8 : Gain  Gain=K_ec_r *(1 + K_act)
  MATLAB Function1 : MATLAB Function  TreatAsAtomicUnit=on
  Sum{,1..8} (9 alike) : Sum  Inputs=|+-
  pdd_ec : Outport
  qdd_ec : Outport  Port=2
  rdd_ec : Outport  Port=3
  wires:
  pd_ref/1 -> Sum/1
  p_ref/1 -> Sum1/1
  Add/1 -> pdd_ec/1
  [p] -> Sum1/2
  [phi] -> Sum2/2
  phi_ref/1 -> Sum2/1
  [pd_f] -> Sum/2
  Sum/1 -> Gain/1  "pd_err"
  Gain/1 -> Add/1
  Sum1/1 -> Gain1/1  "p_err"
  Sum2/1 -> Gain2/1  "phi_err"
  Gain1/1 -> Add/2
  Sum4/1 -> Gain4/1  "q_err"
  [qd_f] -> Sum3/2
  Gain4/1 -> Add1/2
  theta_ref/1 -> Sum5/1
  [theta] -> Sum5/2
  [q] -> Sum4/2
  Gain3/1 -> Add1/1
  q_ref/1 -> Sum4/1
  Add1/1 -> qdd_ec/1
  qd_ref/1 -> Sum3/1
  Sum7/1 -> Gain7/1  "r_err"
  Sum8/1 -> MATLAB Function1/1(pis_e)
  Sum6/1 -> Gain6/1  "rd_err"
  [rd_f] -> Sum6/2
  psi_ref/1 -> Sum8/1
  [psi] -> Sum8/2
  [r] -> Sum7/2
  r_ref/1 -> Sum7/1
  Add2/1 -> rdd_ec/1
  rd_ref/1 -> Sum6/1
  Sum3/1 -> Gain3/1  "qd_err"
  Sum5/1 -> Gain5/1  "theta_err"
  MATLAB Function1/1(psie_w) -> Gain8/1  "psi_err"
  Gain8/1 -> Add2/3
  Gain5/1 -> Add1/3
  Gain2/1 -> Add/3
  Gain7/1 -> Add2/2
  Gain6/1 -> Add2/1

== system B4_quadcopter_model_discrete/Discrete Model - Oversimplified/ERROR CONTROLLER ATTITUDE1 ==
  p_ref : Inport
  q_ref : Inport  Port=2
  r_ref : Inport  Port=3
  phi_ref : Inport  Port=4
  theta_ref : Inport  Port=5
  psi_ref : Inport  Port=6
  Abs : Abs
  Add : Sum  Inputs=+++
  Add1 : Sum  Inputs=+++
  Add2 : Sum  Inputs=+++
  Cumulative Sum : dspmathops/Cumulative Sum  dim=Channels (running sum)  InputProcessing=Columns as channels (frame based)  reset_popup=None  roundingMode=Floor  overflowMode=off  outputDataTypeStr=Inherit: Same as accumulator  outputMin=[]  outputMax=[]  outputLastDataTypeStr=Inherit: Same as accumulator
  Display : Display
  Display1 : Display
  Gain1 : Gain  Gain=K_ec_d_p
  Gain2 : Gain  Gain=K_ec_p
  Gain4 : Gain  Gain=K_ec_d_q
  Gain5 : Gain  Gain=K_ec_q
  Gain7 : Gain  Gain=K_ec_d_r
  Gain8 : Gain  Gain=K_ec_r
  MATLAB Function1 : MATLAB Function  TreatAsAtomicUnit=on
  Mean : dspstat3/Mean  run=off  InputProcessing=Columns as channels (frame based)  reset_popup=None  directionMode=Each column  dimension=1  roiEnable=off  roiType=Rectangles  roiPortion=Entire ROI  roiOutput=Individual statistics for each ROI  roiFlag=off  roundingMode=Floor  overflowMode=off  outputDataTypeStr=Inherit: Same as accumulator  outputMin=[]  outputMax=[]  outputLastDataTypeStr=Inherit: Same as accumulator
  Sum{1..2,4..5,7..8} (6 alike) : Sum  Inputs=|+-
  pd_ec : Outport
  qd_ec : Outport  Port=2
  rd_ec : Outport  Port=3
  wires:
  p_ref/1 -> Sum1/1
  Add/1 -> pd_ec/1
  [p] -> Sum1/2
  [phi] -> Sum2/2
  phi_ref/1 -> Sum2/1
  Sum1/1 -> Gain1/1  "p_err"
  Sum2/1 -> Gain2/1  "phi_err"
  Gain1/1 -> Add/2
  Gain2/1 -> Add/3
  Sum4/1 -> Gain4/1  "q_err"
  Sum5/1 -> Abs/1, Gain5/1  "theta_err"
  Gain4/1 -> Add1/2
  Gain5/1 -> Add1/3
  theta_ref/1 -> Sum5/1
  [theta] -> Sum5/2
  [q] -> Sum4/2
  q_ref/1 -> Sum4/1
  Add1/1 -> qd_ec/1
  Sum7/1 -> Gain7/1  "r_err"
  MATLAB Function1/1(psie_w) -> Gain8/1  "psi_err"
  Gain7/1 -> Add2/2
  Gain8/1 -> Add2/3
  psi_ref/1 -> Sum8/1
  [psi] -> Sum8/2
  [r] -> Sum7/2
  r_ref/1 -> Sum7/1
  Add2/1 -> rd_ec/1
  Sum8/1 -> MATLAB Function1/1(pis_e)
  Cumulative Sum/1 -> Display/1
  Mean/1 -> Display1/1
  Abs/1 -> Mean/1, Cumulative Sum/1  "theta_err_abs"

== system B4_quadcopter_model_discrete/Discrete Model - Oversimplified/INTERNAL REFERENCE MODEL ATTITUDE ==
  phi_cmd : Inport
  theta_cmd : Inport  Port=2
  psi_cmd : Inport  Port=3
  Discrete-Time Integrator{,1..8} (9 alike) : DiscreteIntegrator  SampleTime=sampling_time  ICPrevOutput=DiscIntNeverNeededParam  ICPrevScaledInput=DiscIntNeverNeededParam
  Gain1 : Gain  Gain=K_q_dd
  Gain2 : Gain  Gain=K_p_dd
  Gain3 : Gain  Gain=K_r_dd
  Gain4 : Gain  Gain=K_p_d
  Gain5 : Gain  Gain=K_q_d
  Gain6 : Gain  Gain=K_r_d
  Gain7 : Gain  Gain=K_p
  Gain8 : Gain  Gain=K_q
  Gain9 : Gain  Gain=K_r
  MATLAB Function1 : MATLAB Function  TreatAsAtomicUnit=on
  Sum{1..4,11,16,20..22} (9 alike) : Sum  Inputs=|+-
  pdd_ref : Outport
  qdd_ref : Outport  Port=2
  rdd_ref : Outport  Port=3
  pd_ref : Outport  Port=4
  qd_ref : Outport  Port=5
  rd_ref : Outport  Port=6
  p_ref : Outport  Port=7
  q_ref : Outport  Port=8
  r_ref : Outport  Port=9
  phi_ref : Outport  Port=10
  theta_ref : Outport  Port=11
  psi_ref : Outport  Port=12
  tag scope: p_ref=global, phi_ref=global, psi_ref=global, q_ref=global, r_ref=global, theta_ref=global
  wires:
  Discrete-Time Integrator1/1 -> [theta_ref], theta_ref/1, Sum11/2  "theta_ref"
  Discrete-Time Integrator8/1 -> Sum4/2, Discrete-Time Integrator5/1, rd_ref/1  "rd_ref"
  Discrete-Time Integrator3/1 -> Discrete-Time Integrator2/1, [p_ref], p_ref/1, Sum21/2  "p_ref"
  Discrete-Time Integrator5/1 -> Discrete-Time Integrator/1, [r_ref], r_ref/1, Sum22/2  "r_ref"
  Discrete-Time Integrator4/1 -> Discrete-Time Integrator1/1, [q_ref], q_ref/1, Sum16/2  "q_ref"
  Discrete-Time Integrator7/1 -> Sum3/2, Discrete-Time Integrator4/1, qd_ref/1  "qd_ref"
  Sum21/1 -> Gain4/1
  Sum11/1 -> Gain8/1
  Sum22/1 -> Gain6/1
  Sum16/1 -> Gain5/1
  Discrete-Time Integrator2/1 -> [phi_ref], phi_ref/1, Sum20/2  "phi_ref"
  Sum20/1 -> Gain7/1
  Discrete-Time Integrator6/1 -> Sum2/2, Discrete-Time Integrator3/1, pd_ref/1  "pd_ref"
  phi_cmd/1 -> Sum20/1
  theta_cmd/1 -> Sum11/1
  psi_cmd/1 -> Sum1/1  "psi_cmd"
  Discrete-Time Integrator/1 -> [psi_ref], psi_ref/1, Sum1/2  "psi_ref"
  Sum1/1 -> MATLAB Function1/1(pis_e)  "err"
  Gain4/1 -> Sum2/1
  Gain5/1 -> Sum3/1
  Gain6/1 -> Sum4/1
  Sum2/1 -> Gain2/1
  Sum3/1 -> Gain1/1
  Sum4/1 -> Gain3/1
  Gain2/1 -> Discrete-Time Integrator6/1, pdd_ref/1  "pdd_ref"
  Gain1/1 -> Discrete-Time Integrator7/1, qdd_ref/1  "qdd_ref"
  Gain3/1 -> Discrete-Time Integrator8/1, rdd_ref/1  "rdd_ref"
  Gain7/1 -> Sum21/1
  Gain8/1 -> Sum16/1
  Gain9/1 -> Sum22/1
  MATLAB Function1/1(psie_w) -> Gain9/1  "wrapped_Err"

== system B4_quadcopter_model_discrete/Discrete Model - Oversimplified/INTERNAL REFERENCE MODEL ATTITUDE1 ==
  phi_cmd : Inport
  theta_cmd : Inport  Port=2
  psi_cmd : Inport  Port=3
  Discrete-Time Integrator{,1..5} (6 alike) : DiscreteIntegrator  SampleTime=-1  ICPrevOutput=DiscIntNeverNeededParam  ICPrevScaledInput=DiscIntNeverNeededParam
  Gain4 : Gain  Gain=K_p_d
  Gain5 : Gain  Gain=K_q_d
  Gain6 : Gain  Gain=K_r_d
  Gain7 : Gain  Gain=K_p
  Gain8 : Gain  Gain=K_q
  Gain9 : Gain  Gain=K_r
  MATLAB Function1 : MATLAB Function  TreatAsAtomicUnit=on
  Sum{1,11,16,20..22} (6 alike) : Sum  Inputs=|+-
  pd_ref : Outport
  qd_ref : Outport  Port=2
  rd_ref : Outport  Port=3
  p_ref : Outport  Port=4
  q_ref : Outport  Port=5
  r_ref : Outport  Port=6
  phi_ref : Outport  Port=7
  theta_ref : Outport  Port=8
  psi_ref : Outport  Port=9
  wires:
  Discrete-Time Integrator2/1 -> theta_ref/1, Sum11/2  "theta_ref"
  Gain6/1 -> Discrete-Time Integrator5/1, rd_ref/1  "rd_ref"
  Discrete-Time Integrator/1 -> Discrete-Time Integrator1/1, p_ref/1, Sum21/2  "p_ref"
  Discrete-Time Integrator5/1 -> Discrete-Time Integrator3/1, r_ref/1, Sum22/2  "r_ref"
  Discrete-Time Integrator4/1 -> Discrete-Time Integrator2/1, q_ref/1, Sum16/2  "q_ref"
  Gain5/1 -> Discrete-Time Integrator4/1, qd_ref/1  "qd_ref"
  Sum21/1 -> Gain4/1
  Sum11/1 -> Gain8/1
  Sum22/1 -> Gain6/1
  Sum16/1 -> Gain5/1
  Discrete-Time Integrator1/1 -> phi_ref/1, Sum20/2  "phi_ref"
  Sum20/1 -> Gain7/1
  Gain4/1 -> Discrete-Time Integrator/1, pd_ref/1  "pd_ref"
  phi_cmd/1 -> Sum20/1
  theta_cmd/1 -> Sum11/1
  psi_cmd/1 -> Sum1/1
  Discrete-Time Integrator3/1 -> psi_ref/1, Sum1/2  "psi_ref"
  Sum1/1 -> MATLAB Function1/1(pis_e)
  Gain8/1 -> Sum16/1
  Gain7/1 -> Sum21/1
  Gain9/1 -> Sum22/1
  MATLAB Function1/1(psie_w) -> Gain9/1

== system B4_quadcopter_model_discrete/Tester Block/8-shaped trajectory ==
  Clock : Clock
      settings: Decimation=100
  Constant : Constant  Value=f_8
  Constant1 : Constant  Value=scale_8
  Constant2 : Constant  Value=t_8
  Constant3 : Constant  Value=sampling_time
  MATLAB Function : MATLAB Function  TreatAsAtomicUnit=on
  Switch : Switch  Criteria=u2 > Threshold  Threshold=t_8
  Terminator : Terminator
  XY Graph : Record  FileSettingsInternal="{\"entries\":[{\"content\":{\"excelSettings\":{\"content\":{},\"type\":\"Streamout.ExcelSettings\"}},\"type\":\"Streamout.FileSettingStorage\",\"uuid\":\"e796762b-185b-477d-a421-b293dd71beeb\"}],\"packageUris\":[\"http://schema.mathworks.com/mf0/streamout_blocks/R2020a\"],\"version\":\"1.0\"}"  Layout=[1 1]  SignalsInternal="{\"entries\":[{\"content\":{\"signals\":[]},\"type\":\"RecordBlkView.InputSignals\",\"uuid\":\"715ca310-e917-4639-9881-a7af9902f738\"}],\"packageUris\":[\"http://schema.mathworks.com/mf0/streamout_blocks/R2020a\"],\"version\":\"1.0\"}"  VisualizationBindings="{\"xyplotplugin\":{\"info\":[{\"series\":[],\"subplotID\":1}]}}"  CompatibilityTag=XY
  Zero-Order Hold : ZeroOrderHold  SampleTime=sampling_time
  wires:
  Clock/1 -> Zero-Order Hold/1
  Constant/1 -> MATLAB Function/2(f)
  Constant1/1 -> MATLAB Function/3(scale)
  MATLAB Function/1(x) -> XY Graph/1  "x_traj"
  MATLAB Function/2(y) -> XY Graph/2  "y_traj"
  Constant2/1 -> Switch/1
  Switch/1 -> MATLAB Function/1(t)  "t"
  Zero-Order Hold/1 -> Switch/2, Switch/3
  MATLAB Function/3(phi) -> Terminator/1  "phi_traj"
  Constant3/1 -> MATLAB Function/4(sampling_time)

== system B4_quadcopter_model_discrete/Tester Block/Complementary Filter ==
  y : Inport
  y_model : Inport  Port=2
  Butterworth Lowpass 2nd Order1 : Subsystem
  Butterworth Lowpass 2nd Order2 : Subsystem
  Sum : Sum  Inputs=|++
  Sum1 : Sum  Inputs=|+-
  y_est_no_delay : Outport
  wires:
  y/1 -> Butterworth Lowpass 2nd Order1/1(In)  "y"
  Butterworth Lowpass 2nd Order1/1(Out) -> Sum/1  "y_f"
  Butterworth Lowpass 2nd Order2/1(Out) -> Sum1/2  "y_model_f"
  Sum1/1 -> Sum/2
  y_model/1 -> Butterworth Lowpass 2nd Order2/1(In), Sum1/1  "y_model"
  Sum/1 -> y_est_no_delay/1  "y_est_undelayed"

== system B4_quadcopter_model_discrete/Tester Block/Slowdown Actuator ==
  Discrete Transfer Fcn : DiscreteTransferFcn  Numerator=[0.6 -0.5418]  Denominator=[1 -0.9418]  SampleTime=sampling_time
  Discrete Transfer Fcn1 : DiscreteTransferFcn  Numerator=[0.6 -0.5418]  Denominator=[1 -0.9418]  SampleTime=sampling_time
  Discrete Transfer Fcn2 : DiscreteTransferFcn  Numerator=[0.05824]  Denominator=[1 -0.9418]  SampleTime=sampling_time
  Discrete Transfer Fcn3 : DiscreteTransferFcn  Numerator=[0.05824]  Denominator=[1 -0.9418]  SampleTime=sampling_time
  LTI System : cstblocks/LTI System  sys=tf_des_d  IC=[]
  Scope : Scope  NumInputPorts=2
  Scope1 : Scope  NumInputPorts=2
  Scope2 : Scope  NumInputPorts=3
  Sine Wave : Sin  Frequency=4  SampleTime=0
  Step : Step  SampleTime=0
  Step1 : Step  SampleTime=0
  Sum : Sum  Inputs=|++
  Sum1 : Sum  Inputs=|++
  Transfer Fcn1 : TransferFcn  Numerator=[omega_des]  Denominator=[1 omega_des]
  Transfer Fcn2 : TransferFcn  Numerator=[omega_des]  Denominator=[1 omega_des]
  Transfer Fcn3 : TransferFcn  Numerator=[omega_act]  Denominator=[1 omega_act]
  Transfer Fcn4 : TransferFcn  Numerator=[omega_act]  Denominator=[1 omega_act]
  Transfer Fcn5 : TransferFcn  Numerator=[omega_des]  Denominator=[1 omega_des]
  wires:
  Sine Wave/1 -> Sum1/1, Sum/1
  Sum/1 -> Discrete Transfer Fcn2/1, Discrete Transfer Fcn1/1
  Discrete Transfer Fcn1/1 -> Transfer Fcn4/1
  Discrete Transfer Fcn2/1 -> Sum/2
  Transfer Fcn4/1 -> Scope/1
  Sum1/1 -> Transfer Fcn1/1
  Transfer Fcn1/1 -> Sum1/2, Scope/2  "u_act"
  Transfer Fcn2/1 -> Scope1/2  "u_act"
  Discrete Transfer Fcn/1 -> Transfer Fcn3/1
  Step/1 -> Transfer Fcn2/1, Discrete Transfer Fcn/1
  Transfer Fcn3/1 -> Scope1/1
  Discrete Transfer Fcn3/1 -> Scope2/1
  Step1/1 -> Discrete Transfer Fcn3/1, LTI System/1, Transfer Fcn5/1
  Transfer Fcn5/1 -> Scope2/3  "u_act"
  LTI System/1 -> Scope2/2

== system B4_quadcopter_model_discrete/Tester Block/Tester Actuator State Estimator ==
  Constant1 : Constant  Value=0
  Constant2 : Constant  Value=0
  Constant3 : Constant  Value=0
  Constant5 : Constant  Value=FILT_CUTOFF  SampleTime=sampling_time
  Demux : Demux
  Discrete Transfer Fcn{,1..3} (4 alike) : DiscreteTransferFcn  Numerator=[0.09516]  Denominator=[1 -0.9048]  SampleTime=sampling_time
  Lowpass2 : cstblocks/Linear Parameter Varying/Discrete Varying Lowpass  N=2  w0=0  Ts=sampling_time
      settings: SourceProductBaseCode=CT
  Mux : Mux
  Step : Step  SampleTime=0
  Terminator{,1..3} (4 alike) : Terminator
  wires:
  Demux/3 -> Terminator2/1  "omega_3_est"
  Demux/4 -> Terminator3/1  "omega_4_est"
  Demux/1 -> Terminator/1  "omega_1_est"
  Demux/2 -> Terminator1/1  "omega_2_est"
  Step/1 -> Discrete Transfer Fcn/1  "omega_2_in"
  Constant1/1 -> Discrete Transfer Fcn1/1  "omega_1_in"
  Constant2/1 -> Discrete Transfer Fcn2/1  "omega_3_in"
  Constant3/1 -> Discrete Transfer Fcn3/1  "omega_4_in"
  Constant5/1 -> Lowpass2/2
  Discrete Transfer Fcn3/1 -> Mux/4
  Discrete Transfer Fcn2/1 -> Mux/3
  Discrete Transfer Fcn/1 -> Mux/2
  Discrete Transfer Fcn1/1 -> Mux/1
  Mux/1 -> Lowpass2/1
  Lowpass2/1 -> Demux/1
